simulink model "lstm"  (R2020a)
settings: Solver=FixedStepDiscrete  StartTime=0.0  StopTime=inf  FixedStep=0.002  RelTol=1e-3  EnableMultiTasking=on
libraries: robotlib x2
settings Model: ExtModeTrigDuration=10000  Creator=user  LastModifiedBy=anees
settings SolverCC: PositivePriorityOrder=on
settings DataIOCC: ReturnWorkspaceOutputs=off
settings OptimizationCC: LifeSpan=inf
settings DebuggingCC: ArithmeticOperatorsInVariantConditions=warning
settings SFSimCC: SimUseLocalCustomCode=off  CustomCodeUndefinedFunction=UseInterfaceOnly
settings RTWCC: Description=QUARC Win64 Target  SystemTargetFile=quarc_win64.tlc  TemplateMakefile=quarc_default_tmf  RTWUseLocalCustomCode=off
settings CodeAppCC: StateflowObjectComments=on
settings STFCustomTargetCC: TargetPreCompLibLocation=C:\PROGRA~3\QUARC\lib\2019a\win64\release  TargetLangStandard=C99 (ISO)  ConcurrentExecutionCompliant=on  GRTInterface=on  SystemTargetFile=quarc_win64.tlc
settings GRTTargetCC: TargetPreCompLibLocation=C:\PROGRA~3\QUARC\lib\2019a\win64\release  ParMdlRefBuildCompliant=off  CompOptLevelCompliant=off  CombineOutputUpdateFcns=off  MatFileLogging=off  CPPClassGenCompliant=off  GRTInterface=on  UseToolchainInfoCompliant=off  ExtMode=on  ExtModeMexFile=quarc_comm
settings ConfigComp: CovMetricSettings=dswe

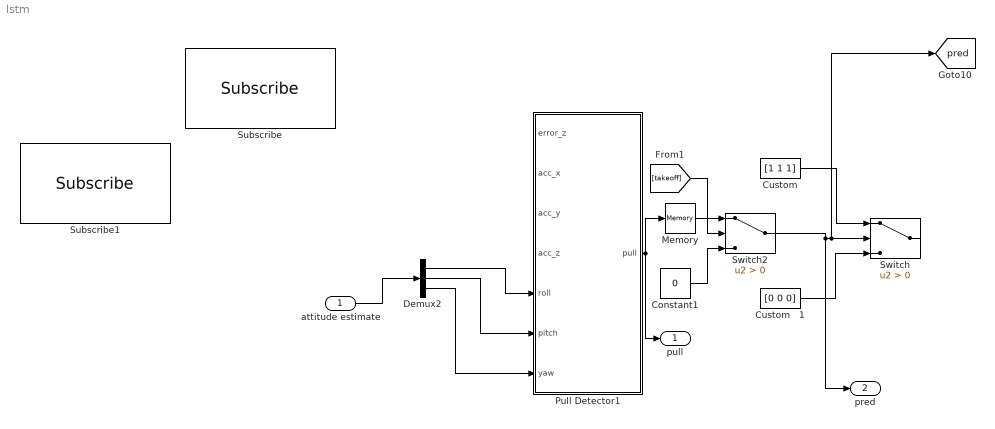
== system lstm ==
  attitude estimate : Inport
  "   Custom   " : Constant  Value=[1 1 1]
  "   Custom   1" : Constant  Value=[0 0 0]
  Constant1 : Constant  Value=0
  Demux2 : Demux  Outputs=3
  Memory : Memory
  Pull Detector1 : Subsystem
  Subscribe : robotlib/Subscribe  topicSource=Select from ROS network  topic=/error_h  messageType=geometry_msgs/Point  sampleTime=-1  messageQueueLength=1
  Subscribe1 : robotlib/Subscribe  topicSource=Select from ROS network  topic=imu  messageType=geometry_msgs/Point  sampleTime=-1  messageQueueLength=1
  Switch : Switch  Criteria=u2 > Threshold
  Switch2 : Switch  Criteria=u2 > Threshold
  "pull " : Outport  VectorParamsAs1DForOutWhenUnconnected=off
  pred : Outport  Port=2  VectorParamsAs1DForOutWhenUnconnected=off
  tag scope: pred=global
  wires:
  ? -> Pull Detector1/1(error_z)
  Memory/1 -> Switch2/1
  attitude estimate/1 -> Demux2/1
  Demux2/3 -> Pull Detector1/7(yaw)
  Constant1/1 -> Switch2/3
  "   Custom   "/1 -> Switch/1
  Switch2/1 -> Switch/2, [pred], pred/1
  Pull Detector1/1(pull) -> Memory/1, "pull "/1
  Demux2/2 -> Pull Detector1/6(pitch)
  [takeoff] -> Switch2/2
  "   Custom   1"/1 -> Switch/3
  Demux2/1 -> Pull Detector1/5(roll)

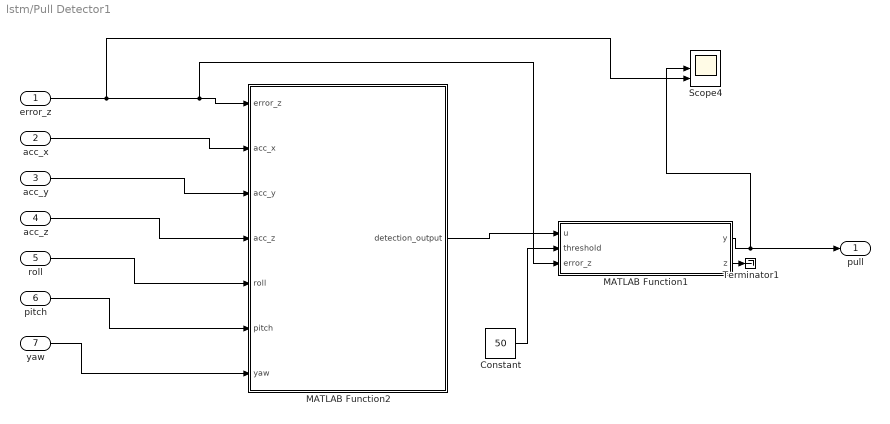
== system lstm/Pull Detector1 ==
  error_z : Inport
  acc_x : Inport  Port=2
  acc_y : Inport  Port=3
  acc_z : Inport  Port=4
  roll : Inport  Port=5
  pitch : Inport  Port=6
  yaw : Inport  Port=7
  Constant : Constant  Value=50  OutDataTypeStr=single
  MATLAB Function1 : MATLAB Function  TreatAsAtomicUnit=on
  MATLAB Function2 : MATLAB Function  TreatAsAtomicUnit=on
  Scope4 : Scope  NumInputPorts=3
  Terminator1 : Terminator
  pull : Outport
  wires:
  roll/1 -> MATLAB Function2/5(roll)
  Constant/1 -> MATLAB Function1/2(threshold)
  acc_x/1 -> MATLAB Function2/2(acc_x)
  acc_y/1 -> MATLAB Function2/3(acc_y)
  acc_z/1 -> MATLAB Function2/4(acc_z)
  pitch/1 -> MATLAB Function2/6(pitch)
  error_z/1 -> Scope4/3, MATLAB Function1/3(error_z), MATLAB Function2/1(error_z)
  MATLAB Function1/1(y) -> Scope4/2, pull/1
  MATLAB Function1/2(z) -> Terminator1/1
  yaw/1 -> MATLAB Function2/7(yaw)
  MATLAB Function2/1(detection_output) -> MATLAB Function1/1(u)

== matlab function lstm/Pull Detector1/MATLAB Function2 ==
  settings: updateMethod=DISCRETE  sampleTime=0.001
  data: error_z input; acc_x input; acc_y input; acc_z input; roll input; pitch input; yaw input; detection_output output
function detection_output  = LSTM(error_z, acc_x, acc_y, acc_z, roll, pitch, yaw)

persistent drone_handover_model
persistent p_01_h_t
persistent p_01_c_t
persistent p_03_h_t
persistent p_03_c_t
persistent scaling_params
persistent buffer
persistent counter
persistent clean_detection

downsample_by = 5;

if isempty(drone_handover_model)
    drone_handover_model = coder.load('Model_2f_norm/drone_handover_model.mat');
    scaling_params = coder.load('Model_2f_norm/Scaling.mat');
    p_01_h_t = single(zeros(1,200));
    p_01_c_t = single(randn(1,200)/10);
    p_03_h_t = single(zeros(1,100));
    p_03_c_t = single(randn(1,100)/10);
    buffer = single(zeros(7,downsample_by));
    counter = 1;
    clean_detection = 0;
end

buffer(1,counter) = error_z;
buffer(2,counter) = acc_x;
buffer(3,counter) = acc_y;
buffer(4,counter) = acc_z;
buffer(5,counter) = roll;
buffer(6,counter) = pitch;
buffer(7,counter) = yaw;

if counter == 5
    counter = 1;
    error_z = mean(buffer(1,:));
    acc_x = mean(buffer(2,:));
    acc_y = mean(buffer(3,:));
    acc_z = mean(buffer(4,:));
    roll = mean(buffer(5,:));
    pitch = mean(buffer(6,:));
    yaw = mean(buffer(7,:));
    % 
    [acc_x_inertial, acc_y_inertial, acc_z_inertial] = R_B2I(roll, pitch, yaw, acc_x, acc_y, acc_z);
    % 
    l2_norm_acc_inertial = sqrt(acc_x_inertial.^2 + acc_y_inertial.^2);
    % 
    % [ori_body_x, ori_body_y, ori_body_z] = R_I2B(roll, pitch, yaw, 0, 0, 1);
    % 
%     l2_norm_ori = sqrt(ori_body_x.^2 + ori_body_y.^2);
%     % 
%     acc_dir = atan2(acc_y_inertial, acc_x_inertial);
%     ori_dir = atan2(ori_body_y, ori_body_x);
%     
%     if abs(acc_dir - ori_dir) <= pi
%         dist_acc_ori = abs(acc_dir - ori_dir);
%     else
%         dist_acc_ori = 2*pi - abs(acc_dir - ori_dir);
%     end
    
    % %%Scaling
    % % X_std = (X - X.min(axis=0)) / (X.max(axis=0) - X.min(axis=0))
    error_z = (error_z - scaling_params.data_Z_params(1)) / (scaling_params.data_Z_params(2)-scaling_params.data_Z_params(1));
    error_z = error_z * 2 - 1;
    l2_norm_acc_inertial = (l2_norm_acc_inertial  - scaling_params.data_L2_norm_inertial_params(1)) / (scaling_params.data_L2_norm_inertial_params(2)-scaling_params.data_L2_norm_inertial_params(1));
    l2_norm_acc_inertial = l2_norm_acc_inertial * 2 - 1;
    %     l2_norm_ori = (l2_norm_ori - scaling_params.data_L2_norm_ori_params(1)) / (scaling_params.data_L2_norm_ori_params(2)-scaling_params.data_L2_norm_ori_params(1));
%     dist_acc_ori = (dist_acc_ori - scaling_params.data_dist_acc_ori_params(1)) / (scaling_params.data_dist_acc_ori_params(2)-scaling_params.data_dist_acc_ori_params(1));
    % 

    input_data = [error_z l2_norm_acc_inertial];

    [detection, p_01_c_t, p_01_h_t, p_03_c_t, p_03_h_t] = model_classify(input_data, ...
                                                                         drone_handover_model, ...
                                                                         p_01_c_t, ...
                                                                         p_01_h_t, ...
                                                                         p_03_c_t, ...
                                                                         p_03_h_t);
                                                                     
    clean_detection = clean(detection, 0.5);
%     clean_detection = double(detection);
end

counter = counter + 1;

% dist_acc_ori_out = dist_acc_ori;
% l2_norm_ori_out = l2_norm_ori;
% l2_norm_acc_out = l2_norm_acc_inertial;
detection_output = double(clean_detection);

% function [detection_output, error_output, l2_output] = LSTM_offline(error_z_, l2_norm_acc_inertial_)
% 
% persistent drone_handover_model
% persistent p_01_h_t
% persistent p_01_c_t
% persistent p_03_h_t
% persistent p_03_c_t
% persistent scaling_params
% persistent buffer
% persistent counter
% persistent clean_detection
% 
% downsample_by = 5;
% 
% if isempty(drone_handover_model)
%     drone_handover_model = coder.load('Model_2f_norm/drone_handover_model.mat');
%     p_01_h_t = single(zeros(1,200));
%     p_01_c_t = single(randn(1,200)/10);
%     p_03_h_t = single(zeros(1,100));
%     p_03_c_t = single(randn(1,100)/10);
%     buffer = single(zeros(7,downsample_by));
%     counter = 1;
%     clean_detection = 0;
% end
% 
% 
% input_data = [error_z_ l2_norm_acc_inertial_];
% 
% [detection, p_01_c_t, p_01_h_t, p_03_c_t, p_03_h_t] = model_classify(input_data, ...
%                                                                      drone_handover_model, ...
%                                                                      p_01_c_t, ...
%                                                                      p_01_h_t, ...
%                                                                      p_03_c_t, ...
%                                                                      p_03_h_t);
% 
% clean_detection = clean(detection, 0.5);
% 
% error_output = error_z_;
% l2_output = l2_norm_acc_inertial_;
% detection_output = double(clean_detection);

== matlab function lstm/Pull Detector1/MATLAB Function1 ==
  settings: updateMethod=DISCRETE  sampleTime=0.001
  data: u input; y output; threshold input; error_z input; z output
function [y, z]= prediction_filter(u, threshold, error_z)

persistent counter_ones
persistent counter_zeros
persistent pull_detected
persistent prev_u
persistent error
persistent prev_error

if isempty(counter_ones)
    counter_ones = 0;
    counter_zeros = 0;
    prev_u = 0;
    error = 0;
    prev_error =0;
end

if u == 1
    counter_ones = counter_ones + 1;
else
    counter_zeros = counter_zeros + 1;     
end

if prev_u == 0 && u == 1
    counter_zeros = 0;
end

if counter_ones > threshold && counter_zeros < threshold
    pull_detected = 1;
else
    pull_detected = 0;
end

if counter_zeros >= threshold
    counter_ones = 0;
end

if pull_detected == 1 && prev_error ==0
    error = error_z;
end
if pull_detected == 0 && prev_error ~= 0
    error = prev_error;
elseif pull_detected == 0 && prev_error == 0
    error =0;
end

prev_error = error;
prev_u = double(u);
z = error;
y = pull_detected;
